simulink subsystem "GyroIntegrator"  (R2021a)
settings: Solver=VariableStepAuto  StartTime=0.0  StopTime=10.0  RelTol=1e-3
undefined symbols (not defined in the file): Ts
libraries: dspmtrx3 x2, attitude_library x2
settings Model: Creator=Laura  LastModifiedBy=Laura

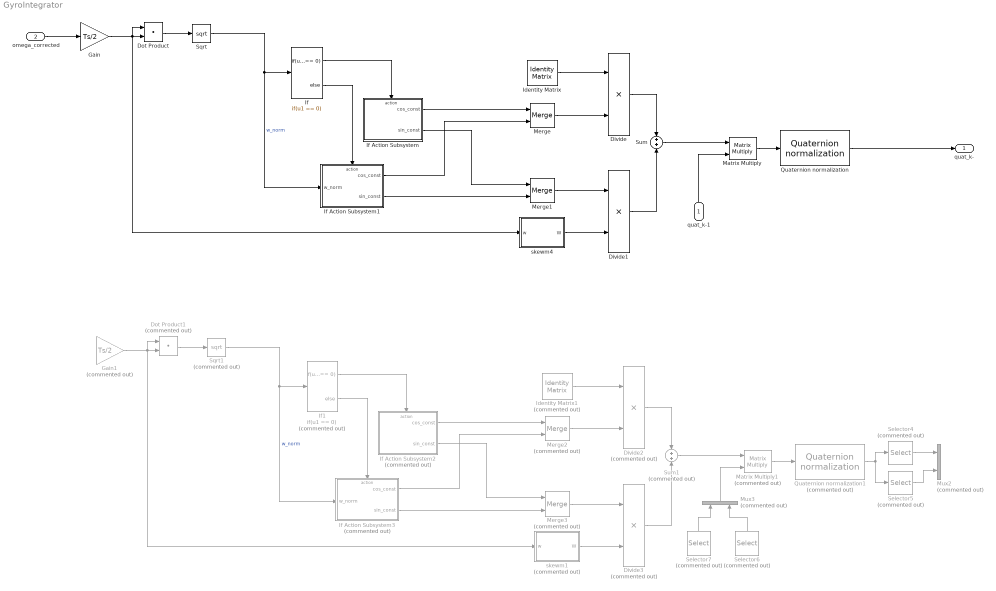
== system GyroIntegrator ==
  quat_k-1 : Inport
  omega_corrected : Inport  Port=2
  Divide : Product  Inputs=**
  Divide1 : Product  Inputs=**
  Divide2 : Product  Commented=on  Inputs=**
  Divide3 : Product  Commented=on  Inputs=**
  Dot Product : DotProduct  InputSameDT=on  OutDataTypeStr=Inherit: Inherit via internal rule
  Dot Product1 : DotProduct  Commented=on  InputSameDT=on  OutDataTypeStr=Inherit: Inherit via internal rule
  Gain : Gain  Gain=Ts/2
  Gain1 : Gain  Commented=on  Gain=Ts/2
  Identity Matrix : dspmtrx3/Identity Matrix  Inherit=off  N=4  Ts=1  dataType=double  isSigned=on  wordLen=16  udDataType=sfix(16)  fracBitsMode=Best precision  numFracBits=15  OutDataTypeStr=double  LastOutDataTypeStr=double
  Identity Matrix1 : dspmtrx3/Identity Matrix  Commented=on  Inherit=off  N=4  Ts=1  dataType=double  isSigned=on  wordLen=16  udDataType=sfix(16)  fracBitsMode=Best precision  numFracBits=15  OutDataTypeStr=double  LastOutDataTypeStr=double
  If : If  IfExpression=u1 == 0
  If Action Subsystem : Subsystem  TreatAsAtomicUnit=on
  If Action Subsystem1 : Subsystem  TreatAsAtomicUnit=on
  If Action Subsystem2 : Subsystem  Commented=on  TreatAsAtomicUnit=on
  If Action Subsystem3 : Subsystem  Commented=on  TreatAsAtomicUnit=on
  If1 : If  Commented=on  IfExpression=u1 == 0
  Matrix Multiply : Product  Multiplication=Matrix(*)
  Matrix Multiply1 : Product  Commented=on  Multiplication=Matrix(*)
  Merge : Merge
  Merge1 : Merge
  Merge2 : Merge  Commented=on
  Merge3 : Merge  Commented=on
  Mux2 : Mux  Commented=on  Inputs=2
  Mux3 : Mux  Commented=on  Inputs=2
  Quaternion normalization : attitude_library/Quaternion normalization  SystemSampleTime=-1  VariantActivationTime=update diagram  Latency=0  AutoFrameSizeCalculation=off
      settings: SourceProductName=Attitude library
  Quaternion normalization1 : attitude_library/Quaternion normalization  Commented=on  SystemSampleTime=-1  VariantActivationTime=update diagram  Latency=0  AutoFrameSizeCalculation=off
      settings: SourceProductName=Attitude library
  Selector4 : Selector  Commented=on  InputPortWidth=4  IndexOptions=Index vector (dialog)  Indices=[4]  OutputSizes=1
  Selector5 : Selector  Commented=on  InputPortWidth=4  IndexOptions=Index vector (dialog)  Indices=[1 2 3]  OutputSizes=1
  Selector6 : Selector  Commented=on  InputPortWidth=4  IndexOptions=Index vector (dialog)  Indices=[1]  OutputSizes=1
  Selector7 : Selector  Commented=on  InputPortWidth=4  IndexOptions=Index vector (dialog)  Indices=[2 3 4]  OutputSizes=1
  Sqrt : Sqrt  SaturateOnIntegerOverflow=on
  Sqrt1 : Sqrt  Commented=on  SaturateOnIntegerOverflow=on
  Sum : Sum
  Sum1 : Sum  Commented=on
  skewm1 : MATLAB Function  Commented=on  TreatAsAtomicUnit=on
  skewm4 : MATLAB Function  TreatAsAtomicUnit=on
  quat_k- : Outport
  wires:
  quat_k-1/1 -> Matrix Multiply/2
  Mux3/1 -> Matrix Multiply1/2
  Selector5/1 -> Mux2/2
  Selector6/1 -> Mux3/2
  Matrix Multiply1/1 -> Quaternion normalization1/1
  Merge3/1 -> Divide3/1
  Selector7/1 -> Mux3/1
  If Action Subsystem2/2(sin_const) -> Merge3/1
  Sum1/1 -> Matrix Multiply1/1
  Merge2/1 -> Divide2/2
  skewm1/1(W) -> Divide3/2
  Divide2/1 -> Sum1/1
  Divide3/1 -> Sum1/2
  Identity Matrix1/1 -> Divide2/1
  If Action Subsystem3/2(sin_const) -> Merge3/2
  If Action Subsystem3/1(cos_const) -> Merge2/2
  If1/2 -> If Action Subsystem3/Action
  If Action Subsystem2/1(cos_const) -> Merge2/1
  Gain1/1 -> skewm1/1(w), Dot Product1/2, Dot Product1/1
  If1/1 -> If Action Subsystem2/Action
  Sqrt1/1 -> If Action Subsystem3/1(w_norm), If1/1  "w_norm"
  Dot Product1/1 -> Sqrt1/1
  Quaternion normalization1/1 -> Selector4/1, Selector5/1
  Selector4/1 -> Mux2/1
  Quaternion normalization/1 -> quat_k-/1
  omega_corrected/1 -> Gain/1
  Gain/1 -> skewm4/1(w), Dot Product/2, Dot Product/1
  Dot Product/1 -> Sqrt/1
  Sqrt/1 -> If Action Subsystem1/1(w_norm), If/1  "w_norm"
  If/1 -> If Action Subsystem/Action
  If/2 -> If Action Subsystem1/Action
  If Action Subsystem/1(cos_const) -> Merge/1
  If Action Subsystem1/1(cos_const) -> Merge/2
  If Action Subsystem/2(sin_const) -> Merge1/1
  If Action Subsystem1/2(sin_const) -> Merge1/2
  Merge/1 -> Divide/2
  Identity Matrix/1 -> Divide/1
  skewm4/1(W) -> Divide1/2
  Merge1/1 -> Divide1/1
  Divide/1 -> Sum/1
  Divide1/1 -> Sum/2
  Sum/1 -> Matrix Multiply/1
  Matrix Multiply/1 -> Quaternion normalization/1

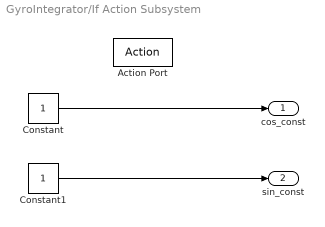
== system GyroIntegrator/If Action Subsystem ==
  Action Port : ActionPort
  Constant : Constant
  Constant1 : Constant
  cos_const : Outport
  sin_const : Outport  Port=2
  wires:
  Constant1/1 -> sin_const/1
  Constant/1 -> cos_const/1

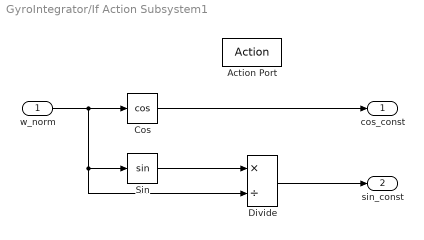
== system GyroIntegrator/If Action Subsystem1 ==
  w_norm : Inport
  Action Port : ActionPort
  Cos : Trigonometry  Operator=cos
  Divide : Product  Inputs=*/
  Sin : Trigonometry
  cos_const : Outport
  sin_const : Outport  Port=2
  wires:
  Cos/1 -> cos_const/1
  Divide/1 -> sin_const/1
  w_norm/1 -> Divide/2, Sin/1, Cos/1
  Sin/1 -> Divide/1

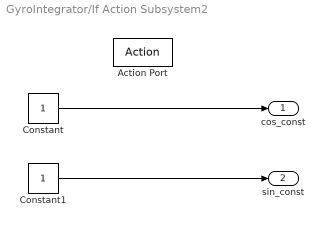
== system GyroIntegrator/If Action Subsystem2 ==
  Action Port : ActionPort
  Constant : Constant
  Constant1 : Constant
  cos_const : Outport
  sin_const : Outport  Port=2
  wires:
  Constant1/1 -> sin_const/1
  Constant/1 -> cos_const/1

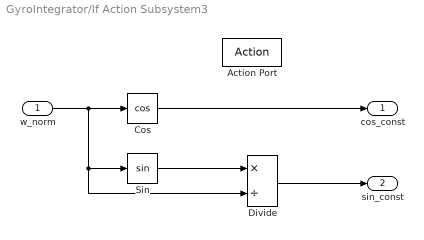
== system GyroIntegrator/If Action Subsystem3 ==
  w_norm : Inport
  Action Port : ActionPort
  Cos : Trigonometry  Operator=cos
  Divide : Product  Inputs=*/
  Sin : Trigonometry
  cos_const : Outport
  sin_const : Outport  Port=2
  wires:
  Cos/1 -> cos_const/1
  Divide/1 -> sin_const/1
  w_norm/1 -> Divide/2, Sin/1, Cos/1
  Sin/1 -> Divide/1

== matlab function GyroIntegrator/skewm1 ==
  data: w input; W output
function W = skewm4(w)
% skewm forms a skew-symmetric 4x4 matrix from a 3x1 vector
%
% INPUT
%              w, 3x1 vector
%
%	OUTPUT
%              W, 4x4 skew-symmetric matrix
%
%%
    W=[  0  w(3)  -w(2)  w(1);
       -w(3)    0  w(1)  w(2);
        w(2) -w(1)   0   w(3);
       -w(1) -w(2) -w(3)    0];
   
end

== matlab function GyroIntegrator/skewm4 ==
  data: w input; W output
function W = skewm4(w)
% skewm forms a skew-symmetric 4x4 matrix from a 3x1 vector
%
% INPUT
%              w, 3x1 vector
%
%	OUTPUT
%              W, 4x4 skew-symmetric matrix
%
%%
%     W=[  0  w(3)  -w(2)  w(1);
%        -w(3)    0  w(1)  w(2);
%         w(2) -w(1)   0   w(3);
%        -w(1) -w(2) -w(3)    0];
   
       W=[  0  -w(1)  -w(2)  -w(3);
          w(1)    0    w(3)  -w(2);
          w(2) -w(3)     0    w(1);
          w(3)  w(2)  -w(1)     0];
   
end
